simulink model "AeroPilotX"  (R2025b)
settings: Solver=ode4  StartTime=0.0  StopTime=30  FixedStep=0.01  RelTol=1e-3
undefined symbols (not defined in the file): SYS
libraries: slpidlib x2
settings Model: Creator=ranadu  LastModifiedBy=ranadu

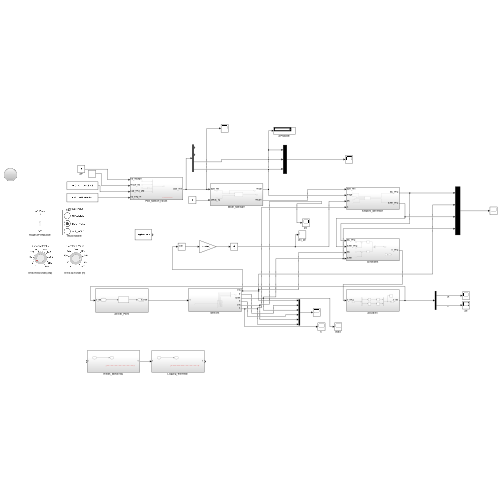
[thumbnail: Simulink's stored preview of the top-level diagram]
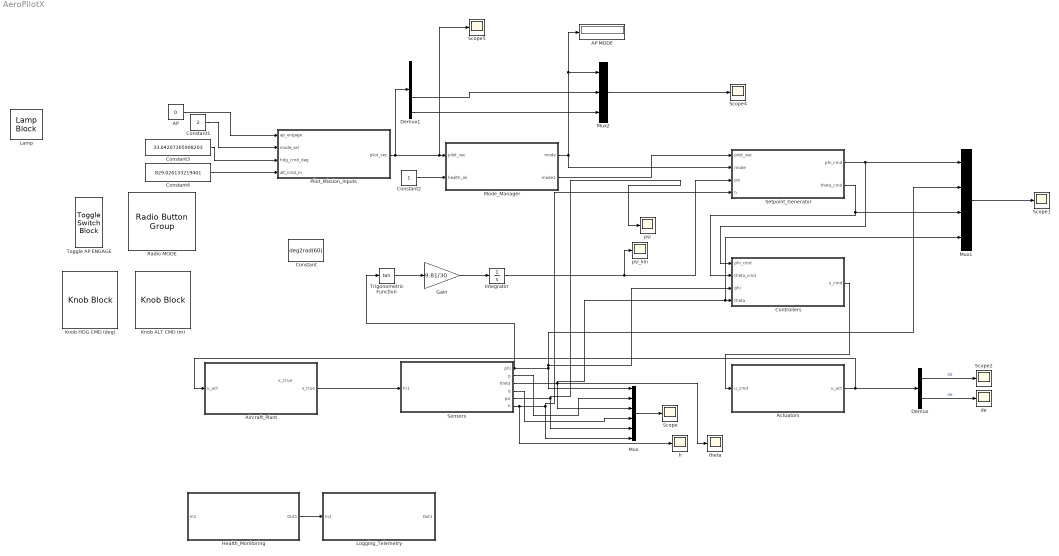
== system AeroPilotX ==
  note: x_true
  AP : Constant  Value=0
  AP MODE : Display
  Actuators : Subsystem  Description=Applies rate limits + saturation. Exposes sat flags + timers.
  Aircraft_Plant : Subsystem  Description=Flight dynamics model (linear first). Truth model (no sensor noise).
  Constant : Constant  Value=deg2rad(60)
  Constant1 : Constant  Value=2
  Constant2 : Constant
  Constant3 : Constant  Value=33.04207305908203
  Constant4 : Constant  Value=829.026133219401
  Controllers : Subsystem  Description=Control laws: inner-loop attitude hold and outer-loop tracking.
  Demux : Demux  Outputs=2
  Demux1 : Demux
  Gain : Gain  Gain=9.81/30
  Health_Monitoring : Subsystem  Description=Evaluates sensors_ok, airspeed_ok, actuator_ok; triggers FAILSAFE conditions.
  Integrator : Integrator
  Knob ALT CMD (m) : KnobBlock  ScaleMax=1000
  Knob HDG CMD (deg) : KnobBlock  ScaleMax=360
  Lamp : LampBlock  LabelPosition=Hide  DefaultColor=[192.0, 192.0, 192.0]
  Logging_Telemetry : Subsystem  Description=Logs signals for validation/plots. Must not feed back into control.
  Mode_Manager : Subsystem  Description=Selects mode (MANUAL/STAB/ALT/HDG/NAV/FAILSAFE) using health + pilot commands.
  Mux : Mux  Inputs=6
  Mux1 : Mux
  Mux2 : Mux  Inputs=3
  Pilot_Mission_Inputs : Subsystem  Description=Pilot buttons and mission setpoints. No control logic.
  Radio MODE : RadioButtonGroup  SelectedLabel=HDG_HOLD  ButtonGroupName=Group
  Scope{,1..2,4..5} (5 alike) : Scope
      Scope settings: ActiveDisplayYMinimum=-1  ActiveDisplayYMaximum=1  DataLoggingVariableName=ScopeData2
      Scope1 settings: ActiveDisplayYMinimum=-0.49087385212340517  ActiveDisplayYMaximum=0.054541539124822784  DataLoggingVariableName=ScopeData3
      Scope2 settings: ActiveDisplayYMinimum=-1  ActiveDisplayYMaximum=1  DataLoggingVariableName=ScopeData4
      Scope4 settings: ActiveDisplayYMinimum=-1  ActiveDisplayYMaximum=1  DataLoggingVariableName=ScopeData6
      Scope5 settings: ActiveDisplayYMinimum=-1  ActiveDisplayYMaximum=1  DataLoggingVariableName=ScopeData7
  Sensors : Subsystem  Description=Adds noise/bias/dropouts. Provides measured states + validity flags.
  Setpoint_Generator : Subsystem  Description=Maps mode + commands into attitude references (phi_cmd, theta_cmd, etc.).
  Toggle AP ENGAGE : ToggleSwitchBlock
  Trigonometric Function : Trigonometry  Operator=tan
  de : Scope
      settings: ActiveDisplayYMinimum=-1  ActiveDisplayYMaximum=1  DataLoggingVariableName=ScopeData5
  h : Scope
      settings: ActiveDisplayYMinimum=-1  ActiveDisplayYMaximum=1  DataLoggingVariableName=ScopeData9
  psi : Scope
      settings: ActiveDisplayYMinimum=-1  ActiveDisplayYMaximum=1  DataLoggingVariableName=ScopeData8
  psi_kin : Scope
      settings: ActiveDisplayYMinimum=-1  ActiveDisplayYMaximum=1  DataLoggingVariableName=ScopeData11
  theta : Scope
      settings: ActiveDisplayYMinimum=-1  ActiveDisplayYMaximum=1  DataLoggingVariableName=ScopeData10
  wires:
  Health_Monitoring/1(Out1) -> Logging_Telemetry/1(In1)
  Controllers/1(u_cmd) -> Actuators/1(u_cmd)
  Actuators/1(u_act) -> Aircraft_Plant/1(u_act), Demux/1
  Constant1/1 -> Pilot_Mission_Inputs/2(mode_sel)
  AP/1 -> Pilot_Mission_Inputs/1(ap_engage)
  Constant4/1 -> Pilot_Mission_Inputs/4(alt_cmd_m)
  Constant3/1 -> Pilot_Mission_Inputs/3(hdg_cmd_deg)
  Constant2/1 -> Mode_Manager/2(health_ok)
  Mode_Manager/1(mode) -> Mux2/1, AP MODE/1, Setpoint_Generator/2(mode)
  Setpoint_Generator/1(phi_cmd) -> Mux1/1, Controllers/1(phi_cmd)
  Setpoint_Generator/2(theta_cmd) -> Mux1/3, Controllers/2(theta_cmd)
  Pilot_Mission_Inputs/1(pilot_vec) -> Scope5/1, Mode_Manager/1(pilot_vec), Demux1/1
  Aircraft_Plant/1(x_true) -> Sensors/1(In1)
  Sensors/1(phi) -> Trigonometric Function/1, Mux1/2, Controllers/3(phi), Mux/1
  Sensors/3(theta) -> theta/1, Mux1/4, Controllers/4(theta), Mux/3
  Sensors/5(psi) -> psi/1, Mux/5
  Sensors/6(h) -> h/1, Setpoint_Generator/4(h), Mux/6
  Sensors/4(q) -> Mux/4
  Sensors/2(p) -> Mux/2
  Mux/1 -> Scope/1
  Mux1/1 -> Scope1/1
  Demux/2 -> de/1  "de"
  Demux/1 -> Scope2/1  "da"
  Demux1/4 -> Mux2/3
  Demux1/3 -> Mux2/2
  Mux2/1 -> Scope4/1
  Mode_Manager/2(mode1) -> Setpoint_Generator/1(pilot_vec)
  Trigonometric Function/1 -> Gain/1
  Gain/1 -> Integrator/1
  Integrator/1 -> psi_kin/1, Setpoint_Generator/3(psi)

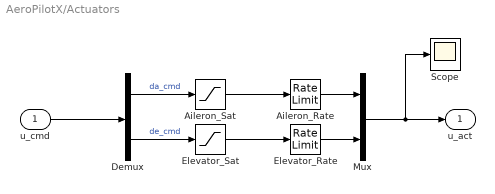
== system AeroPilotX/Actuators ==
  u_cmd : Inport
  Aileron_Rate : RateLimiter  RisingSlewLimit=deg2rad(80)  FallingSlewLimit=-deg2rad(80)  SampleTimeMode=inherited
  Aileron_Sat : Saturate  UpperLimit=deg2rad(20)  LowerLimit=-deg2rad(20)
  Demux : Demux  Outputs=2
  Elevator_Rate : RateLimiter  RisingSlewLimit=deg2rad(60)  FallingSlewLimit=-deg2rad(60)  SampleTimeMode=inherited
  Elevator_Sat : Saturate  UpperLimit=deg2rad(25)  LowerLimit=-deg2rad(25)
  Mux : Mux  Inputs=2
  Scope : Scope
      settings: ActiveDisplayYMinimum=-1  ActiveDisplayYMaximum=1
  u_act : Outport
  wires:
  u_cmd/1 -> Demux/1
  Aileron_Rate/1 -> Mux/1
  Elevator_Rate/1 -> Mux/2
  Elevator_Sat/1 -> Elevator_Rate/1
  Aileron_Sat/1 -> Aileron_Rate/1
  Demux/1 -> Aileron_Sat/1  "da_cmd"
  Demux/2 -> Elevator_Sat/1  "de_cmd"
  Mux/1 -> Scope/1, u_act/1

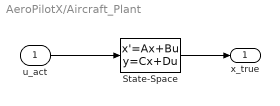
== system AeroPilotX/Aircraft_Plant ==
  u_act : Inport
  State-Space : StateSpace  A=SYS.A  B=SYS.B  C=SYS.C  D=SYS.D  InitialCondition=SYS.x0
  x_true : Outport
  wires:
  State-Space/1 -> x_true/1
  u_act/1 -> State-Space/1

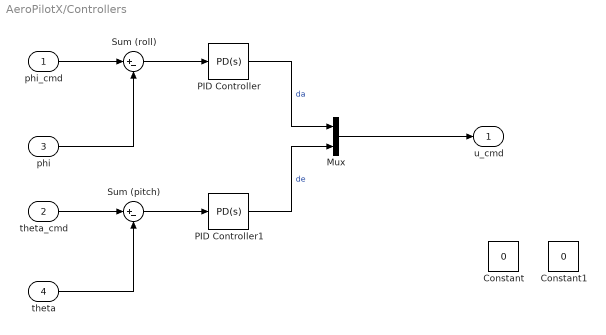
== system AeroPilotX/Controllers ==
  phi_cmd : Inport
  theta_cmd : Inport  Port=2
  phi : Inport  Port=3
  theta : Inport  Port=4
  Constant : Constant  Value=0
  Constant1 : Constant  Value=0
  Mux : Mux  Inputs=2
  PID Controller : slpidlib/PID Controller  Controller=PD  Form=Parallel  TimeDomain=Continuous-time  UseExternalTs=off  SampleTime=-1  IntegratorMethod=Forward Euler  FilterMethod=Forward Euler  ControllerParametersSource=internal  P=2  I=1  UseKiTs=off  D=0.5  UseExternalDerivativeSource=off  N=100  UseFilter=on  TunerSelectOption=Transfer Function Based (PID Tuner App)  InitialConditionSource=internal  InitialConditionForIntegrator=0  InitialConditionForFilter=0  DifferentiatorICPrevScaledInput=0  ExternalReset=none  TrackingMode=off  Kt=1  LimitOutput=off  SatLimitsSource=internal  UpperSaturationLimit=inf  LowerSaturationLimit=-inf  LinearizeAsGain=on  AntiWindupMode=none  Kb=1  LimitIntegrator=off  UpperIntegratorSaturationLimit=inf  LowerIntegratorSaturationLimit=-inf  POutMin=[]  POutMax=[]  IOutMin=[]  IOutMax=[]  DOutMin=[]  DOutMax=[]  NOutMin=[]  NOutMax=[]  SumOutMin=[]  SumOutMax=[]  SaturationOutMin=[]  SaturationOutMax=[]  PParamMin=[]  PParamMax=[]  IParamMin=[]  IParamMax=[]  DParamMin=[]  DParamMax=[]  NParamMin=[]  NParamMax=[]  KbParamMin=[]  KbParamMax=[]  KtParamMin=[]  KtParamMax=[]  KbOutMin=[]  KbOutMax=[]  KtOutMin=[]  KtOutMax=[]  IntegratorOutMin=[]  IntegratorOutMax=[]  FilterOutMin=[]  FilterOutMax=[]  SumI1OutMin=[]  SumI1OutMax=[]  SumI2OutMin=[]  SumI2OutMax=[]  SumI3OutMin=[]  SumI3OutMax=[]  SumI4OutMin=[]  SumI4OutMax=[]  SumDOutMin=[]  SumDOutMax=[]  DifferentiatorOutMin=[]  DifferentiatorOutMax=[]  FilterDiffOutCoefMin=[]  FilterDiffOutCoefMax=[]  ReciprocalOutMin=[]  ReciprocalOutMax=[]  SumDenOutMin=[]  SumDenOutMax=[]  SumNumOutMin=[]  SumNumOutMax=[]  DivideOutMin=[]  DivideOutMax=[]  UdiffTsProdOutMin=[]  UdiffTsProdOutMax=[]  NTsProdOutMin=[]  NTsProdOutMax=[]  UintegralTsProdOutMin=[]  UintegralTsProdOutMax=[]  UngainTsProdOutMin=[]  UngainTsProdOutMax=[]  ClampingZeroOutDataTypeStr=Inherit: Inherit via back propagation  ClampingZeroOutMin=[]  ClampingZeroOutMax=[]  FilterDenConstantOutDataTypeStr=Inherit: Inherit via back propagation  FilterDenConstantOutMin=[]  FilterDenConstantOutMax=[]  PCopyOutDataTypeStr=Inherit: Inherit via back propagation  PCopyOutMin=[]  PCopyOutMax=[]  NCopyOutDataTypeStr=Inherit: Inherit via back propagation  NCopyOutMin=[]  NCopyOutMax=[]  IntegratorContinuousStateAttributes=''  IntegratorStateMustResolveToSignalObject=off  IntegratorRTWStateStorageClass=Auto  FilterContinuousStateAttributes=''  FilterStateMustResolveToSignalObject=off  FilterRTWStateStorageClass=Auto  ParallelPVariant=InternalParameters  IdealPVariant=Disabled  IVariant=Disabled  DVariant=InternalParameters  IntegratorVariant=Disabled  SatVariant=Disabled  AWVariant=Disabled  PCopyVariant=Disabled  TRVariant=Disabled  FdbkBlocksVariant=Forward  IdealPFdbkVariant=Disabled  SatFdbkVariant=Disabled  DerivativeFilterVariant=ContFilter  NVariant=InternalParameters  NCopyVariant=Disabled  FilterICVariant=InternalICsFilter  IntegratorICVariant=Disabled  ExternalResetVariant=Disabled  TRSumVariant=Passthrough  SumFdbkVariant=Disabled  SumVariant=Sum_PD  TsampFilterVariant=InternalTs  TsampNgainVariant=Passthrough  TsampIntegralVariant=Disabled_SignalSpec  ExternalSaturationOutDataTypeStr=Inherit: Same as second input  DerivativeSourceVariant=ErrorSignal  PreIntVariant=InternalPreInt
  PID Controller1 : slpidlib/PID Controller  Controller=PD  Form=Parallel  TimeDomain=Continuous-time  UseExternalTs=off  SampleTime=-1  IntegratorMethod=Forward Euler  FilterMethod=Forward Euler  ControllerParametersSource=internal  P=2.5  I=1  UseKiTs=off  D=0.6  UseExternalDerivativeSource=off  N=100  UseFilter=on  TunerSelectOption=Transfer Function Based (PID Tuner App)  InitialConditionSource=internal  InitialConditionForIntegrator=0  InitialConditionForFilter=0  DifferentiatorICPrevScaledInput=0  ExternalReset=none  TrackingMode=off  Kt=1  LimitOutput=off  SatLimitsSource=internal  UpperSaturationLimit=inf  LowerSaturationLimit=-inf  LinearizeAsGain=on  AntiWindupMode=none  Kb=1  LimitIntegrator=off  UpperIntegratorSaturationLimit=inf  LowerIntegratorSaturationLimit=-inf  POutMin=[]  POutMax=[]  IOutMin=[]  IOutMax=[]  DOutMin=[]  DOutMax=[]  NOutMin=[]  NOutMax=[]  SumOutMin=[]  SumOutMax=[]  SaturationOutMin=[]  SaturationOutMax=[]  PParamMin=[]  PParamMax=[]  IParamMin=[]  IParamMax=[]  DParamMin=[]  DParamMax=[]  NParamMin=[]  NParamMax=[]  KbParamMin=[]  KbParamMax=[]  KtParamMin=[]  KtParamMax=[]  KbOutMin=[]  KbOutMax=[]  KtOutMin=[]  KtOutMax=[]  IntegratorOutMin=[]  IntegratorOutMax=[]  FilterOutMin=[]  FilterOutMax=[]  SumI1OutMin=[]  SumI1OutMax=[]  SumI2OutMin=[]  SumI2OutMax=[]  SumI3OutMin=[]  SumI3OutMax=[]  SumI4OutMin=[]  SumI4OutMax=[]  SumDOutMin=[]  SumDOutMax=[]  DifferentiatorOutMin=[]  DifferentiatorOutMax=[]  FilterDiffOutCoefMin=[]  FilterDiffOutCoefMax=[]  ReciprocalOutMin=[]  ReciprocalOutMax=[]  SumDenOutMin=[]  SumDenOutMax=[]  SumNumOutMin=[]  SumNumOutMax=[]  DivideOutMin=[]  DivideOutMax=[]  UdiffTsProdOutMin=[]  UdiffTsProdOutMax=[]  NTsProdOutMin=[]  NTsProdOutMax=[]  UintegralTsProdOutMin=[]  UintegralTsProdOutMax=[]  UngainTsProdOutMin=[]  UngainTsProdOutMax=[]  ClampingZeroOutDataTypeStr=Inherit: Inherit via back propagation  ClampingZeroOutMin=[]  ClampingZeroOutMax=[]  FilterDenConstantOutDataTypeStr=Inherit: Inherit via back propagation  FilterDenConstantOutMin=[]  FilterDenConstantOutMax=[]  PCopyOutDataTypeStr=Inherit: Inherit via back propagation  PCopyOutMin=[]  PCopyOutMax=[]  NCopyOutDataTypeStr=Inherit: Inherit via back propagation  NCopyOutMin=[]  NCopyOutMax=[]  IntegratorContinuousStateAttributes=''  IntegratorStateMustResolveToSignalObject=off  IntegratorRTWStateStorageClass=Auto  FilterContinuousStateAttributes=''  FilterStateMustResolveToSignalObject=off  FilterRTWStateStorageClass=Auto  ParallelPVariant=InternalParameters  IdealPVariant=Disabled  IVariant=Disabled  DVariant=InternalParameters  IntegratorVariant=Disabled  SatVariant=Disabled  AWVariant=Disabled  PCopyVariant=Disabled  TRVariant=Disabled  FdbkBlocksVariant=Forward  IdealPFdbkVariant=Disabled  SatFdbkVariant=Disabled  DerivativeFilterVariant=ContFilter  NVariant=InternalParameters  NCopyVariant=Disabled  FilterICVariant=InternalICsFilter  IntegratorICVariant=Disabled  ExternalResetVariant=Disabled  TRSumVariant=Passthrough  SumFdbkVariant=Disabled  SumVariant=Sum_PD  TsampFilterVariant=InternalTs  TsampNgainVariant=Passthrough  TsampIntegralVariant=Disabled_SignalSpec  ExternalSaturationOutDataTypeStr=Inherit: Same as second input  DerivativeSourceVariant=ErrorSignal  PreIntVariant=InternalPreInt
  Sum (pitch) : Sum  Inputs=|+-
  Sum (roll) : Sum  Inputs=|+-
  u_cmd : Outport
  wires:
  phi/1 -> Sum (roll)/2
  Sum (roll)/1 -> PID Controller/1
  theta/1 -> Sum (pitch)/2
  Sum (pitch)/1 -> PID Controller1/1
  PID Controller/1 -> Mux/1  "da"
  PID Controller1/1 -> Mux/2  "de"
  Mux/1 -> u_cmd/1
  theta_cmd/1 -> Sum (pitch)/1
  phi_cmd/1 -> Sum (roll)/1

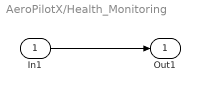
== system AeroPilotX/Health_Monitoring ==
  In1 : Inport
  Out1 : Outport
  wires:
  ? -> ?
  In1/1 -> Out1/1

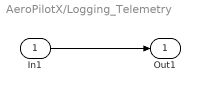
== system AeroPilotX/Logging_Telemetry ==
  In1 : Inport
  Out1 : Outport
  wires:
  ? -> ?
  In1/1 -> Out1/1

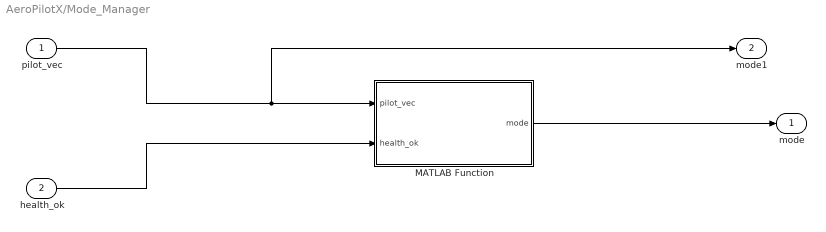
== system AeroPilotX/Mode_Manager ==
  pilot_vec : Inport  PortDimensions=4
  health_ok : Inport  Port=2
  MATLAB Function : MATLAB Function  TreatAsAtomicUnit=on
  mode : Outport
  mode1 : Outport  Port=2
  wires:
  pilot_vec/1 -> MATLAB Function/1(pilot_vec), mode1/1
  health_ok/1 -> MATLAB Function/2(health_ok)
  MATLAB Function/1(mode) -> mode/1

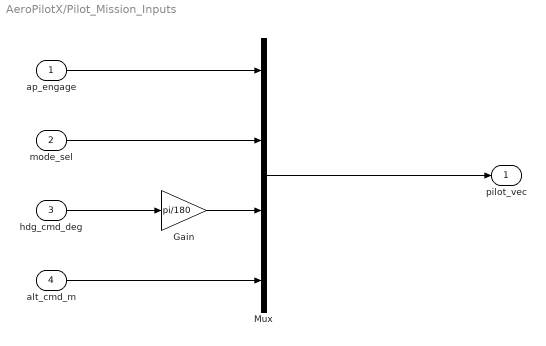
== system AeroPilotX/Pilot_Mission_Inputs ==
  ap_engage : Inport
  mode_sel : Inport  Port=2
  hdg_cmd_deg : Inport  Port=3
  alt_cmd_m : Inport  Port=4
  Gain : Gain  Gain=pi/180
  Mux : Mux
  pilot_vec : Outport  PortDimensions=4
  wires:
  ? -> ?
  hdg_cmd_deg/1 -> Gain/1
  ap_engage/1 -> Mux/1
  Gain/1 -> Mux/3
  mode_sel/1 -> Mux/2
  alt_cmd_m/1 -> Mux/4
  Mux/1 -> pilot_vec/1

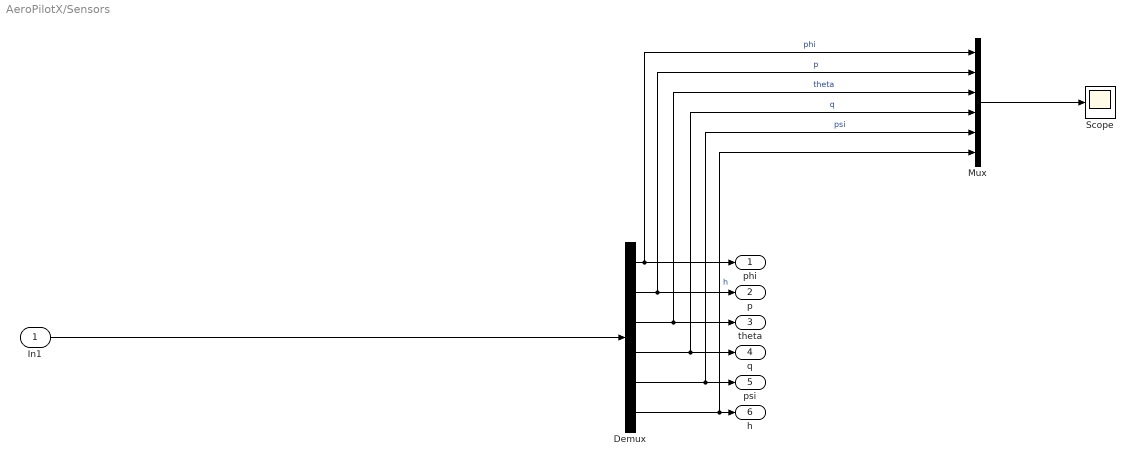
== system AeroPilotX/Sensors ==
  In1 : Inport
  Demux : Demux  Outputs=6
  Mux : Mux  Inputs=6
  Scope : Scope
  phi : Outport
  p : Outport  Port=2
  theta : Outport  Port=3
  q : Outport  Port=4
  psi : Outport  Port=5
  h : Outport  Port=6
  wires:
  Demux/5 -> Mux/5, psi/1  "psi"
  Demux/1 -> Mux/1, phi/1  "phi"
  Demux/4 -> Mux/4, q/1  "q"
  Demux/3 -> Mux/3, theta/1  "theta"
  Demux/2 -> Mux/2, p/1  "p"
  Demux/6 -> Mux/6, h/1  "h"
  Mux/1 -> Scope/1
  In1/1 -> Demux/1

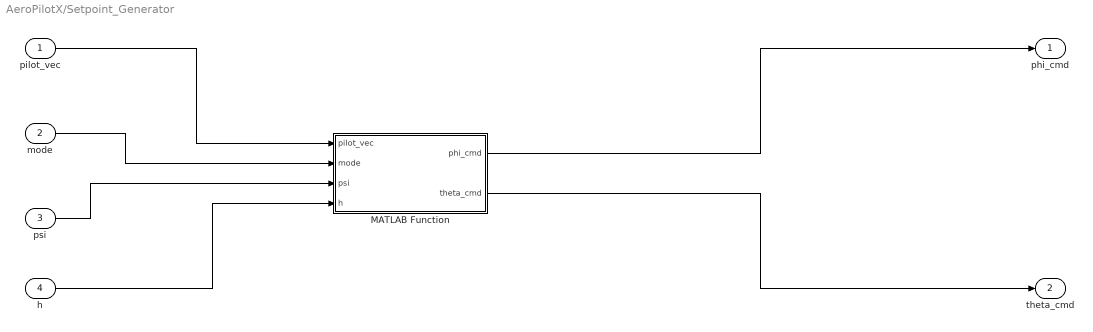
== system AeroPilotX/Setpoint_Generator ==
  pilot_vec : Inport  PortDimensions=4
  mode : Inport  Port=2
  psi : Inport  Port=3
  h : Inport  Port=4
  MATLAB Function : MATLAB Function  TreatAsAtomicUnit=on
  phi_cmd : Outport
  theta_cmd : Outport  Port=2
  wires:
  pilot_vec/1 -> MATLAB Function/1(pilot_vec)
  mode/1 -> MATLAB Function/2(mode)
  psi/1 -> MATLAB Function/3(psi)
  h/1 -> MATLAB Function/4(h)
  MATLAB Function/1(phi_cmd) -> phi_cmd/1
  MATLAB Function/2(theta_cmd) -> theta_cmd/1

== matlab function AeroPilotX/Setpoint_Generator/MATLAB Function ==
  data: pilot_vec input; phi_cmd output; mode input; psi input; h input; theta_cmd output
function [phi_cmd, theta_cmd] = sp_gen(pilot_vec, mode, psi, h)
% SP_GEN — Autopilot Setpoint Generator (Guidance Layer)
%
% Inputs:
%   pilot_vec = [ap_engage; mode_sel; hdg_cmd_rad; alt_cmd_m]
%   mode      = 0 MANUAL
%               1 STABILIZE
%               2 HDG_HOLD
%               3 ALT_HOLD
%   psi       = current heading (rad)
%   h         = current altitude (m)
%
% Outputs:
%   phi_cmd   = commanded roll angle (rad)
%   theta_cmd = commanded pitch angle (rad)

% -------------------------------------------------
% Unpack pilot commands
% -------------------------------------------------
ap_engage = pilot_vec(1);
hdg_cmd   = pilot_vec(3);   % rad
alt_cmd   = pilot_vec(4);   % m

% -------------------------------------------------
% Guidance gains (NOT controller gains)
% -------------------------------------------------
K_hdg_guidance = 1.5;    % rad roll per rad heading error
K_alt_guidance = 0.02;   % rad pitch per meter altitude error

% -------------------------------------------------
% Command limits (aircraft-level)
% -------------------------------------------------
phi_max   = deg2rad(25);   % max bank command
theta_max = deg2rad(15);   % max pitch command

% -------------------------------------------------
% Deadbands (reduce steady-state chatter)
% -------------------------------------------------
hdg_deadband = deg2rad(1);  % 1 deg heading deadband
alt_deadband = 1.0;         % 1 m altitude deadband

% -------------------------------------------------
% Defaults (safe)
% -------------------------------------------------
phi_cmd   = 0;
theta_cmd = 0;

% -------------------------------------------------
% AP disengaged → zero commands
% -------------------------------------------------
if ap_engage < 0.5
    return;
end

% -------------------------------------------------
% Mode-based logic
% -------------------------------------------------
if mode == 1
    % STABILIZE
    % Hold wings level and zero pitch
    phi_cmd   = 0;
    theta_cmd = 0;

elseif mode == 2
    % HDG_HOLD
    % Roll command from heading error

    % Heading error wrapped to [-pi, pi]
    hdg_err = hdg_cmd - psi;
    hdg_err = atan2(sin(hdg_err), cos(hdg_err));

    % Deadband
    if abs(hdg_err) < hdg_deadband
        hdg_err = 0;
    end

    % Guidance law
    phi_cmd = saturate( ...
        K_hdg_guidance * hdg_err, ...
        -phi_max, phi_max );

    theta_cmd = 0;

elseif mode == 3
    % ALT_HOLD
    % Pitch command from altitude error

    alt_err = alt_cmd - h;

    % Deadband
    if abs(alt_err) < alt_deadband
        alt_err = 0;
    end

    % Guidance law
    theta_cmd = saturate( ...
        K_alt_guidance * alt_err, ...
        -theta_max, theta_max );

    phi_cmd = 0;

else
    % MANUAL / FAILSAFE
    phi_cmd   = 0;
    theta_cmd = 0;
end

end

% -------------------------------------------------
% Helper: saturation
% -------------------------------------------------
function y = saturate(u, lo, hi)
y = min(max(u, lo), hi);
end

== matlab function AeroPilotX/Mode_Manager/MATLAB Function ==
  data: pilot_vec input; mode output; health_ok input
function mode = mode_logic(pilot_vec, health_ok)

ap_engage = pilot_vec(1);
mode_sel  = pilot_vec(2);

mode = 0; % MANUAL (double)

if ap_engage < 0.5
    mode = 0;
    return;
end

if health_ok < 0.5
    mode = 5; % FAILSAFE (reserved)
    return;
end

% Allowed modes: 1..3
if mode_sel < 1
    mode = 1;
elseif mode_sel > 3
    mode = 3;
else
    mode = mode_sel;
end
end
